simulink model "TTECTrA_block"  (Simulink 8.0)
settings: Solver=ode45  StartTime=0.0  StopTime=10.0  RelTol=1e-3
values from neighbouring files (symbols this model uses):
  DWS = setup_TTECTrA_block(DWS,inputs)    [simFromTTECTrA.m]
undefined symbols (not defined in the file or in its folder): DiscIntNeverNeededParam
libraries: simulink_extras x1, simulink x1
settings Model: Creator=azinneck  LastModifiedBy=jcsank
settings DebuggingCC: FcnCallInpInsideContextMsg=EnableAllAsWarning
settings CodeAppCC: CustomSymbolStrType=$N$R$M_T  InternalIdentifier=Shortened
settings GRTTargetCC: CombineOutputUpdateFcns=off  GRTInterface=on

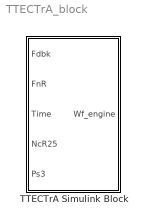
== system TTECTrA_block ==
  "TTECTrA Simulink Block " : Subsystem

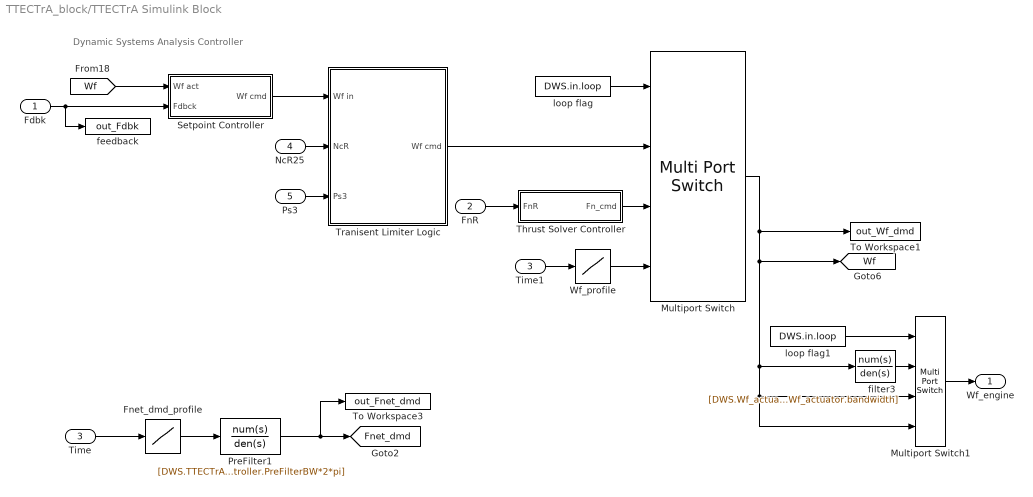
== system TTECTrA_block/TTECTrA Simulink Block  ==
  note: Dynamic Systems Analysis Controller
  Fdbk : Inport
  "FnR " : Inport  Port=2
  Time : Inport  Port=3
  NcR25 : Inport  Port=4
  Ps3 : Inport  Port=5
  Fnet_dmd_profile : Lookup  InputValues=DWS.in.t_vec  Table=DWS.in.FT_dmd  SampleTime=DWS.in.Ts_cont
  Multiport Switch : MultiPortSwitch
  Multiport Switch1 : MultiPortSwitch
  PreFilter1 : TransferFcn  Numerator=[DWS.TTECTrA_controller.PreFilterBW*2*pi]  Denominator=[1 DWS.TTECTrA_controller.PreFilterBW*2*pi]
  Setpoint Controller : Subsystem
  Thrust Solver Controller : Subsystem
  Time1 : InportShadow  Port=3
  To Workspace1 : ToWorkspace  VariableName=out_Wf_dmd  SampleTime=-1
  To Workspace3 : ToWorkspace  VariableName=out_Fnet_dmd  SampleTime=-1
  Tranisent Limiter Logic : Subsystem
  Wf_profile : Lookup  InputValues=DWS.in.t_vec  Table=DWS.in.wf_vec  SampleTime=DWS.in.Ts_cont
  feedback : ToWorkspace  VariableName=out_Fdbk  SampleTime=-1
  filter3 : TransferFcn  Numerator=[DWS.Wf_actuator.bandwidth]  Denominator=[1 DWS.Wf_actuator.bandwidth]
  loop flag : Constant  Value=DWS.in.loop
  loop flag1 : Constant  Value=DWS.in.loop
  Wf_engine : Outport
  tag scope: Fnet_dmd=global, Wf=global
  wires:
  loop flag/1 -> Multiport Switch/1
  [Wf] -> Setpoint Controller/1(Wf act)
  Fdbk/1 -> feedback/1, Setpoint Controller/2(Fdbck)
  "FnR "/1 -> Thrust Solver Controller/1(FnR)
  Time/1 -> Fnet_dmd_profile/1
  Thrust Solver Controller/1(Fn_cmd) -> Multiport Switch/3
  Wf_profile/1 -> Multiport Switch/4
  Time1/1 -> Wf_profile/1
  Multiport Switch1/1 -> Wf_engine/1
  Multiport Switch/1 -> To Workspace1/1, filter3/1, Multiport Switch1/4, Multiport Switch1/3, [Wf]
  loop flag1/1 -> Multiport Switch1/1
  Setpoint Controller/1(Wf cmd) -> Tranisent Limiter Logic/1(Wf in)
  Tranisent Limiter Logic/1(Wf cmd) -> Multiport Switch/2
  NcR25/1 -> Tranisent Limiter Logic/2(NcR)
  Ps3/1 -> Tranisent Limiter Logic/3(Ps3)
  Fnet_dmd_profile/1 -> PreFilter1/1
  PreFilter1/1 -> To Workspace3/1, [Fnet_dmd]
  filter3/1 -> Multiport Switch1/2

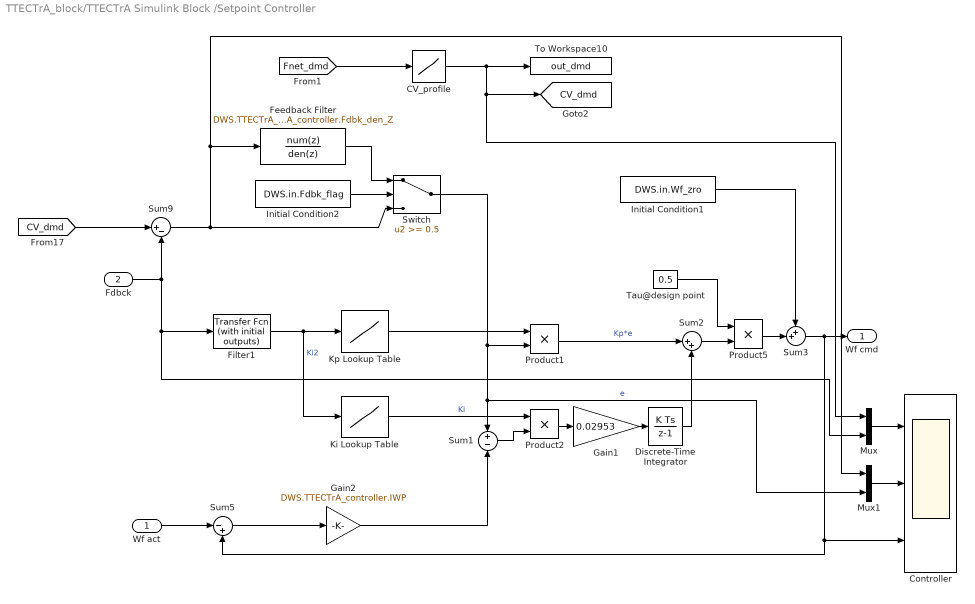
== system TTECTrA_block/TTECTrA Simulink Block /Setpoint Controller ==
  Wf act : Inport
  Fdbck : Inport  Port=2
  CV_profile : Lookup  InputValues=DWS.TTECTrA_setpoints.FT_bkpt  Table=DWS.TTECTrA_setpoints.SP  SampleTime=DWS.in.Ts_cont
  Controller : Scope  NumInputPorts=3
      settings: YMin=1~-0.3~0  YMax=1.9~0.25~5
  Discrete-Time Integrator : DiscreteIntegrator  SampleTime=DWS.in.Ts_cont  ICPrevOutput=DiscIntNeverNeededParam  ICPrevScaledInput=DiscIntNeverNeededParam
  Feedback Filter : DiscreteTransferFcn  Numerator=DWS.TTECTrA_controller.Fdbk_num_Z  Denominator=DWS.TTECTrA_controller.Fdbk_den_Z  SampleTime=DWS.in.Ts_cont
  Filter1 : simulink_extras/Additional Linear/Transfer Fcn (with initial outputs)  N=[1]  D=[0.1 1]  Y0=0.24  U0=0.24
  Gain1 : Gain  Gain=0.02953
  Gain2 : Gain  Gain=DWS.TTECTrA_controller.IWP
  Initial Condition1 : Constant  Value=DWS.in.Wf_zro
  Initial Condition2 : Constant  Value=DWS.in.Fdbk_flag
  Ki Lookup Table : Lookup_n-D  NumberOfTableDimensions=1  BreakpointsForDimension1=DWS.TTECTrA_controller.Fdbk  Table=DWS.TTECTrA_controller.I_gain  SampleTime=DWS.in.Ts_cont  RndMeth=Simplest  InputSameDT=on
  Kp Lookup Table : Lookup_n-D  NumberOfTableDimensions=1  BreakpointsForDimension1=DWS.TTECTrA_controller.Fdbk  Table=DWS.TTECTrA_controller.P_gain  SampleTime=DWS.in.Ts_cont  RndMeth=Simplest  InputSameDT=on
  Mux : Mux  Inputs=2
  Mux1 : Mux  Inputs=2
  Product1 : Product  SampleTime=DWS.in.Ts_cont  RndMeth=Zero
  Product2 : Product  SampleTime=DWS.in.Ts_cont  RndMeth=Zero
  Product5 : Product  RndMeth=Zero
  Sum1 : Sum  Inputs=+|-
  Sum2 : Sum  Inputs=|++  SampleTime=DWS.in.Ts_cont
  Sum3 : Sum  Inputs=++|  SampleTime=DWS.in.Ts_cont
  Sum5 : Sum  Inputs=|-+  SampleTime=DWS.in.Ts_cont
  Sum9 : Sum  Inputs=|+-  SampleTime=DWS.in.Ts_cont
  Switch : Switch  Threshold=0.5
  Tau@design point : Constant  Value=0.5
  To Workspace10 : ToWorkspace  VariableName=out_dmd  SampleTime=-1
  Wf cmd : Outport
  tag scope: CV_dmd=global
  wires:
  Tau@design point/1 -> Product5/1
  Product1/1 -> Sum2/1  "Kp*e"
  Product2/1 -> Gain1/1
  Sum9/1 -> Mux1/1, Feedback Filter/1, Switch/3
  [CV_dmd] -> Sum9/1
  Wf act/1 -> Sum5/1
  Sum5/1 -> Gain2/1
  Switch/1 -> Product1/2, Mux1/2, Sum1/1  "e"
  Sum1/1 -> Product2/2
  Sum2/1 -> Product5/2
  Gain2/1 -> Sum1/2
  Sum3/1 -> Wf cmd/1, Controller/3, Sum5/2
  Initial Condition1/1 -> Sum3/1
  Product5/1 -> Sum3/2
  Gain1/1 -> Discrete-Time Integrator/1
  Discrete-Time Integrator/1 -> Sum2/2
  Ki Lookup Table/1 -> Product2/1  "Ki"
  Fdbck/1 -> Mux/2, Filter1/1, Sum9/2
  CV_profile/1 -> Mux/1, [CV_dmd], To Workspace10/1
  [Fnet_dmd] -> CV_profile/1
  Kp Lookup Table/1 -> Product1/1
  Filter1/1 -> Ki Lookup Table/1, Kp Lookup Table/1  "Ki2"
  Initial Condition2/1 -> Switch/2
  Feedback Filter/1 -> Switch/1
  Mux/1 -> Controller/1
  Mux1/1 -> Controller/2

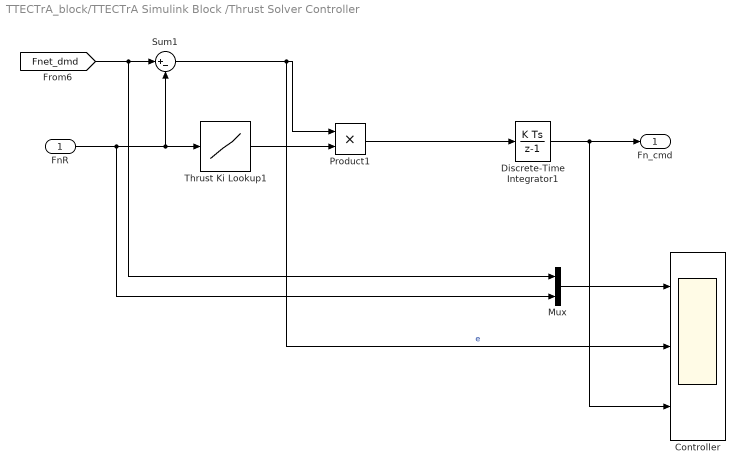
== system TTECTrA_block/TTECTrA Simulink Block /Thrust Solver Controller ==
  FnR : Inport
  Controller : Scope  NumInputPorts=3
      settings: YMin=0~-35000~2.6  YMax=35000~5000~3.05  SaveName=ScopeData3
  Discrete-Time Integrator1 : DiscreteIntegrator  InitialCondition=DWS.in.Wf_zro  SampleTime=DWS.in.Ts_cont  ICPrevOutput=DiscIntNeverNeededParam  ICPrevScaledInput=DiscIntNeverNeededParam
  Mux : Mux  Inputs=2
  Product1 : Product  SampleTime=DWS.in.Ts_cont  RndMeth=Zero
  Sum1 : Sum  Inputs=|+-  SampleTime=DWS.in.Ts_cont
  Thrust Ki Lookup1 : Lookup_n-D  NumberOfTableDimensions=1  BreakpointsForDimension1=[500 10000 20000 30000 40000]  Table="[.005  .005 .0035 .0035 .0035]*.01"  SampleTime=DWS.in.Ts_cont  RndMeth=Simplest  InputSameDT=on
  Fn_cmd : Outport
  wires:
  FnR/1 -> Mux/2, Sum1/2, Thrust Ki Lookup1/1
  [Fnet_dmd] -> Mux/1, Sum1/1
  Discrete-Time Integrator1/1 -> Fn_cmd/1, Controller/3
  Product1/1 -> Discrete-Time Integrator1/1
  Sum1/1 -> Product1/1, Controller/2  "e"
  Thrust Ki Lookup1/1 -> Product1/2
  Mux/1 -> Controller/1

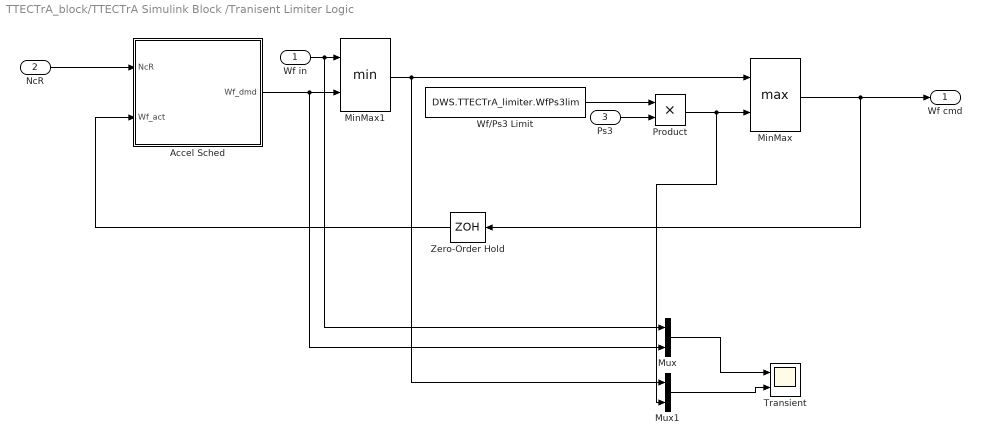
== system TTECTrA_block/TTECTrA Simulink Block /Tranisent Limiter Logic ==
  Wf in : Inport
  NcR : Inport  Port=2
  Ps3 : Inport  Port=3
  Accel Sched : Subsystem
  MinMax : MinMax  Function=max  Inputs=2
  MinMax1 : MinMax  Inputs=2
  Mux : Mux  Inputs=2
  Mux1 : Mux  Inputs=2
  Product : Product  RndMeth=Zero
  Transient : Scope  NumInputPorts=2
      settings: YMin=-5~-5  YMax=5~5
  Wf/Ps3 Limit : Constant  Value=DWS.TTECTrA_limiter.WfPs3lim
  Zero-Order Hold : ZeroOrderHold  SampleTime=DWS.in.Ts_cont
  Wf cmd : Outport
  wires:
  Ps3/1 -> Product/2
  Wf/Ps3 Limit/1 -> Product/1
  Wf in/1 -> Mux/1, MinMax1/1
  MinMax1/1 -> Mux1/1, MinMax/1
  NcR/1 -> Accel Sched/1(NcR)
  Accel Sched/1(Wf_dmd) -> Mux/2, MinMax1/2
  MinMax/1 -> Zero-Order Hold/1, Wf cmd/1
  Zero-Order Hold/1 -> Accel Sched/2(Wf_act)
  Mux/1 -> Transient/1
  Mux1/1 -> Transient/2
  Product/1 -> Mux1/2, MinMax/2

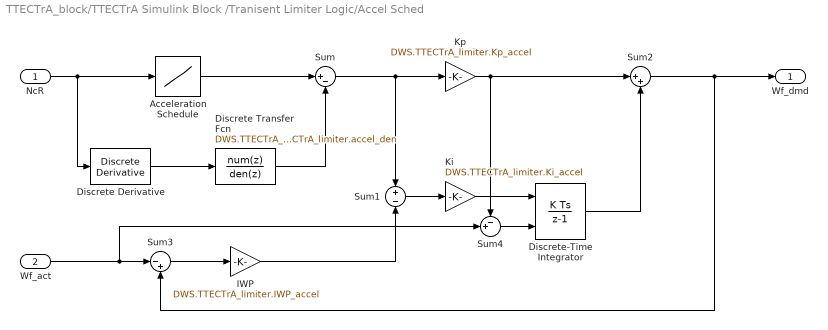
== system TTECTrA_block/TTECTrA Simulink Block /Tranisent Limiter Logic/Accel Sched ==
  NcR : Inport
  Wf_act : Inport  Port=2
  Acceleration Schedule : Lookup  InputValues=DWS.TTECTrA_limiter.Nc_sched  Table=DWS.TTECTrA_limiter.Ncdot_sched
  Discrete Derivative : simulink/Discrete/Discrete Derivative  gainval=1.0  ICPrevScaledInput=DWS.in.Nc_zro/DWS.in.Ts_cont  InputProcessing=Inherited  OutMin=[]  OutMax=[]  OutDataType=fixdt(1, 16)  OutScaling=2^-10  DoSatur=off
  Discrete Transfer Fcn : DiscreteTransferFcn  Numerator=DWS.TTECTrA_limiter.accel_num  Denominator=DWS.TTECTrA_limiter.accel_den  SampleTime=DWS.in.Ts_cont
  Discrete-Time Integrator : DiscreteIntegrator  InitialConditionSource=external  SampleTime=DWS.in.Ts_cont  ICPrevOutput=DiscIntNeverNeededParam  ICPrevScaledInput=DiscIntNeverNeededParam
  IWP : Gain  Gain=DWS.TTECTrA_limiter.IWP_accel
  Ki : Gain  Gain=DWS.TTECTrA_limiter.Ki_accel
  Kp : Gain  Gain=DWS.TTECTrA_limiter.Kp_accel
  Sum : Sum  Inputs=|+-
  Sum1 : Sum  Inputs=+|-
  Sum2 : Sum  Inputs=|++
  Sum3 : Sum  Inputs=|-+
  Sum4 : Sum  Inputs=-+|
  Wf_dmd : Outport
  wires:
  NcR/1 -> Discrete Derivative/1, Acceleration Schedule/1
  Discrete Derivative/1 -> Discrete Transfer Fcn/1
  Acceleration Schedule/1 -> Sum/1
  Discrete Transfer Fcn/1 -> Sum/2
  Sum/1 -> Sum1/1, Kp/1
  Sum1/1 -> Ki/1
  Kp/1 -> Sum2/1, Sum4/1
  Sum2/1 -> Sum3/2, Wf_dmd/1
  Ki/1 -> Discrete-Time Integrator/1
  Discrete-Time Integrator/1 -> Sum2/2
  IWP/1 -> Sum1/2
  Sum3/1 -> IWP/1
  Wf_act/1 -> Sum4/2, Sum3/1
  Sum4/1 -> Discrete-Time Integrator/2
